simulink model "bpsk_receiver"  (R2020a)
settings: Solver=VariableStepAuto  StartTime=0.0  StopTime=10000/3.2e6  RelTol=1e-3
InitFcn:
  | setup_bpsk_receiver
undefined symbols (not defined in the file): AXI4, designMultirateFIR, fir_bbuf, Lite, tx_data, xlfda_numerator
libraries: xbsIndex_r4 x367, hdlsllib x15, dspmlti4 x8, xrbsSSR_Library x6, dspswit3 x4, dspsigops x2, commrandsrc3 x1, simulink x1
(part 3 of 4)

== system bpsk_receiver/Coarse Frequency Synchronisation/NCO ==
  Offset In : Inport
  AddSub : xbsIndex_r4/AddSub  mode=Addition  use_carryin=off  use_carryout=off  en=off  latency=0  precision=User Defined  arith_type=Unsigned  n_bits=41  bin_pt=41-10  quantization=Truncate  overflow=Wrap  use_behavioral_HDL=off  hw_selection=Fabric  pipelined=off  dbl_ovrd=off  block_type=addsub
  CMult : xbsIndex_r4/CMult  const=1024/(12.8e6)  gui_display_data_type=Fixed-point  const_n_bits=i+b  const_bin_pt=b  float_type=Single  exp_bits=8  fraction_bits=24  en=off  latency=1  precision=User Defined  arith_type="Signed  (2's comp)"  n_bits=n+b  bin_pt=b  quantization=Truncate  overflow=Saturate  use_behavioral_HDL=off  mem_type=Distributed RAM  pipeline=off  dbl_ovrd=off  block_type=cmult
  Convert4 : xbsIndex_r4/Convert  gui_display_data_type=Fixed-point  arith_type=Unsigned  n_bits=10  bin_pt=0  float_type=Single  exp_bits=8  fraction_bits=24  quantization=Truncate  overflow=Wrap  en=off  latency=0  pipeline=off  dbl_ovrd=off  block_type=convert
  Delay2 : xbsIndex_r4/Delay  rst=off  infoeditControl=Selection of Reset will increase slice count due to use of real FFs and instead of SRLs  en=off  latency=1  reg_retiming=off  dbl_ovrd=off  block_type=delay
  Sin_ROM : xbsIndex_r4/ROM  depth=1024  initVector=sin(pi*(0:1024-1)/(1024/2))  distributed_mem=Block RAM  rst=off  init_reg=0  en=off  latency=1  gui_display_data_type=Fixed-point  arith_type="Signed  (2's comp)"  n_bits=L  bin_pt=L-2  preci_type=Single  exp_width=8  frac_width=24  optimize=Area  use_rpm=on  dbl_ovrd=off  simulation_type=fast_sim  block_type=sprom
  cos_ROM : xbsIndex_r4/ROM  depth=1024  initVector=cos(pi*(0:1024-1)/(1024/2))  distributed_mem=Block RAM  rst=off  init_reg=0  en=off  latency=1  gui_display_data_type=Fixed-point  arith_type="Signed  (2's comp)"  n_bits=L  bin_pt=L-2  preci_type=Single  exp_width=8  frac_width=24  optimize=Area  use_rpm=on  dbl_ovrd=off  simulation_type=fast_sim  block_type=sprom
  cos : Outport  VectorParamsAs1DForOutWhenUnconnected=off
  sin : Outport  Port=2  VectorParamsAs1DForOutWhenUnconnected=off
  wires:
  cos_ROM/1 -> cos/1
  Sin_ROM/1 -> sin/1
  Convert4/1 -> cos_ROM/1, Sin_ROM/1
  CMult/1 -> AddSub/2
  Delay2/1 -> AddSub/1
  Offset In/1 -> CMult/1
  AddSub/1 -> Delay2/1, Convert4/1

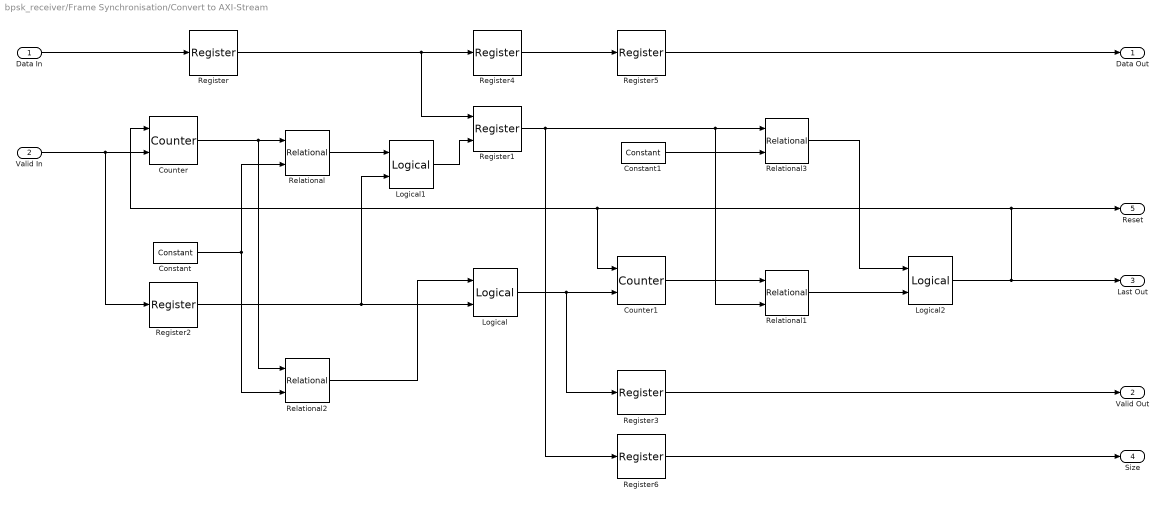
== system bpsk_receiver/Frame Synchronisation/Convert to AXI-Stream ==
  Data In : Inport
  Valid In : Inport  Port=2
  Constant : xbsIndex_r4/Constant  const=1.0  gui_display_data_type=Fixed-point  arith_type=Unsigned  n_bits=1  bin_pt=0  preci_type=Single  exp_width=8  frac_width=24  explicit_period=off  period=1  equ=P=C  opselect=C  inp2=PCIN>>17  opr=+  inp1=P  carry=CIN  dbl_ovrd=off  block_type=constant
  Constant1 : xbsIndex_r4/Constant  const=0  gui_display_data_type=Fixed-point  arith_type=Unsigned  n_bits=1  bin_pt=0  preci_type=Single  exp_width=8  frac_width=24  explicit_period=off  period=1  equ=P=C  opselect=C  inp2=PCIN>>17  opr=+  inp1=P  carry=CIN  dbl_ovrd=off  block_type=constant
  Counter : xbsIndex_r4/Counter  cnt_type=Free Running  cnt_to=Inf  operation=Up  start_count=0  cnt_by_val=1  arith_type=Unsigned  n_bits=32  bin_pt=0  load_pin=off  rst=on  en=on  explicit_period=off  period=1  use_behavioral_HDL=off  implementation=Fabric  dbl_ovrd=off  block_type=counter
  Counter1 : xbsIndex_r4/Counter  cnt_type=Free Running  cnt_to=Inf  operation=Up  start_count=0  cnt_by_val=1  arith_type=Unsigned  n_bits=32  bin_pt=0  load_pin=off  rst=on  en=on  explicit_period=off  period=1  use_behavioral_HDL=off  implementation=Fabric  dbl_ovrd=off  block_type=counter
  Logical : xbsIndex_r4/Logical  logical_function=AND  inputs=2  en=off  latency=1  precision=Full  arith_type=Unsigned  n_bits=16  bin_pt=0  align_bp=on  dbl_ovrd=off  block_type=logical
  Logical1 : xbsIndex_r4/Logical  logical_function=AND  inputs=2  en=off  latency=0  precision=Full  arith_type=Unsigned  n_bits=16  bin_pt=0  align_bp=on  dbl_ovrd=off  block_type=logical
  Logical2 : xbsIndex_r4/Logical  logical_function=AND  inputs=2  en=off  latency=0  precision=Full  arith_type=Unsigned  n_bits=16  bin_pt=0  align_bp=on  dbl_ovrd=off  block_type=logical
  Register{,2..6} (6 alike) : xbsIndex_r4/Register  init=0  rst=off  en=off  dbl_ovrd=off  block_type=register
  Register1 : xbsIndex_r4/Register  init=0  rst=off  en=on  dbl_ovrd=off  block_type=register
  Relational : xbsIndex_r4/Relational  mode=a=b  op_type=Bool  en=off  latency=0  dbl_ovrd=off  block_type=relational
  Relational1 : xbsIndex_r4/Relational  mode=a>=b  op_type=Bool  en=off  latency=0  dbl_ovrd=off  block_type=relational
  Relational2 : xbsIndex_r4/Relational  mode=a>b  op_type=Bool  en=off  latency=0  dbl_ovrd=off  block_type=relational
  Relational3 : xbsIndex_r4/Relational  mode=a!=b  op_type=Bool  en=off  latency=0  dbl_ovrd=off  block_type=relational
  Data Out : Outport  VectorParamsAs1DForOutWhenUnconnected=off
  Valid Out : Outport  Port=2  VectorParamsAs1DForOutWhenUnconnected=off
  Last Out : Outport  Port=3  VectorParamsAs1DForOutWhenUnconnected=off
  Size : Outport  Port=4  VectorParamsAs1DForOutWhenUnconnected=off
  Reset : Outport  Port=5  VectorParamsAs1DForOutWhenUnconnected=off
  wires:
  Register6/1 -> Size/1
  Logical2/1 -> Last Out/1, Reset/1, Counter1/1, Counter/1
  Relational1/1 -> Logical2/2
  Relational3/1 -> Logical2/1
  Constant1/1 -> Relational3/2
  Logical1/1 -> Register1/2
  Relational/1 -> Logical1/1
  Relational2/1 -> Logical/1
  Constant/1 -> Relational2/2, Relational/2
  Register5/1 -> Data Out/1
  Register4/1 -> Register5/1
  Register3/1 -> Valid Out/1
  Register2/1 -> Logical/2, Logical1/2
  Register1/1 -> Relational1/2, Relational3/1, Register6/1
  Counter1/1 -> Relational1/1
  Logical/1 -> Counter1/2, Register3/1
  Register/1 -> Register1/1, Register4/1
  Data In/1 -> Register/1
  Counter/1 -> Relational/1, Relational2/1
  Valid In/1 -> Counter/2, Register2/1

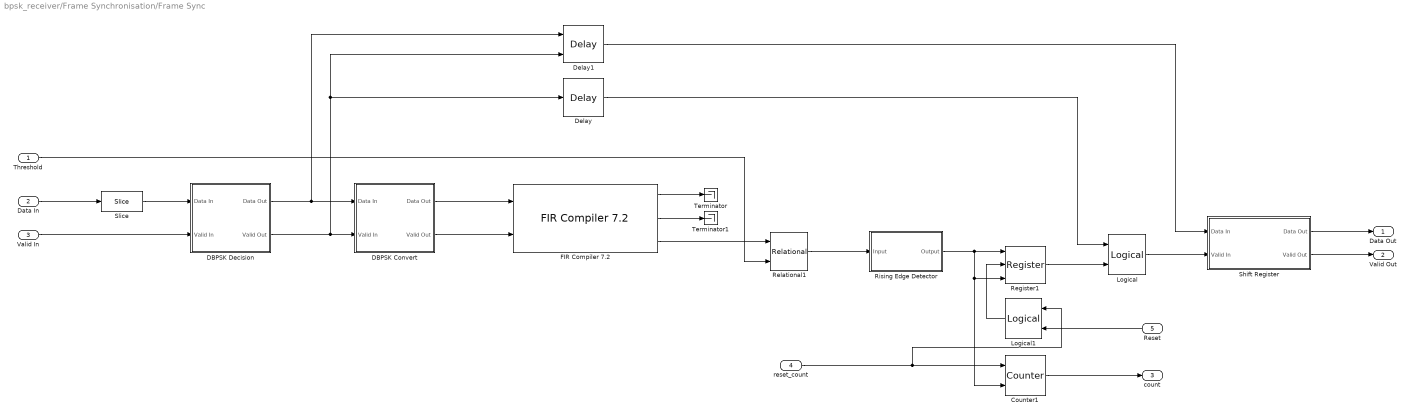
== system bpsk_receiver/Frame Synchronisation/Frame Sync ==
  Threshold : Inport
  Data In : Inport  Port=2
  Valid In : Inport  Port=3
  reset_count : Inport  Port=4
  Reset : Inport  Port=5
  Counter1 : xbsIndex_r4/Counter  cnt_type=Free Running  cnt_to=Inf  operation=Up  start_count=0  cnt_by_val=1  arith_type=Unsigned  n_bits=32  bin_pt=0  load_pin=off  rst=on  en=on  explicit_period=off  period=1  use_behavioral_HDL=off  implementation=Fabric  dbl_ovrd=off  block_type=counter
  DBPSK Convert : Subsystem
  DBPSK Decision : Subsystem
  Delay : xbsIndex_r4/Delay  rst=off  infoeditControl=Selection of Reset will increase slice count due to use of real FFs and instead of SRLs  en=off  latency=2  reg_retiming=off  dbl_ovrd=off  block_type=delay
  Delay1 : xbsIndex_r4/Delay  rst=off  infoeditControl=Selection of Reset will increase slice count due to use of real FFs and instead of SRLs  en=on  latency=2  reg_retiming=off  dbl_ovrd=off  block_type=delay
  "FIR Compiler 7.2 " : xbsIndex_r4/FIR Compiler 7.2   coefficientvector=fliplr(double(fir_bbuf))  coefficient_sets=1  coefficient_reload=off  filter_type=Single_Rate  rate_change_type=Integer  interpolation_rate=1  decimation_rate=1  zero_pack_factor=1  channel_sequence=Basic  number_channels=1  pattern_list='P4-0,P4-1,P4-2,P4-3,P4-4'  number_paths=1  ratespecification=Maximum_Possible  sampleperiod=40  hardwareoversamplingrate=1  coefficient_sign=Signed  quantization=Integer_Coefficients  coefficient_width=2  bestprecision=off  coefficient_fractional_bits=0  coefficient_structure=Inferred  output_rounding_mode=Full_Precision  output_width=22  filter_architecture=Systolic_Multiply_Accumulate  optimization_goal=Area  optimization_list='None'  data_buffer_type=Automatic  coefficient_buffer_type=Automatic  input_buffer_type=Automatic  output_buffer_type=Automatic  preference_for_other_storage=Automatic  multi_column_support=Automatic  columnconfig='39'  inter_column_pipe_length=4  data_has_tlast=Not_Required  m_data_has_tready=off  s_data_has_fifo=off  s_data_has_tuser=Not_Required  m_data_has_tuser=Not_Required  s_config_sync_mode=On_Vector  s_config_method=Single  num_reload_slots=1  has_aclken=on  has_aresetn=off  infoeditControl=ARESETn must be asserted for a minimum of 2 cycles  reset_data_vector=on  trim_axipin_name=on  simulation_type=hybrid_sim  simulation_model=sysgen:xfirv7_2_cmodel  data_path_portlist={ 's_axis_data_tdata', 'm_axis_data_tdata' }  passband_min=0.0  passband_max=0.5  stopband_min=0.5  stopband_max=1.0  filter_selection=1  gui_behaviour='Sysgen_GUI'  data_sign=Signed  data_width=16  data_fractional_bits=0  data_tuser_width=1  wrapper_available=true  ip_wrap_arbitrary_binary_point=true  ip_name=FIR Compiler  ip_version=7.2  dsptool_ready=true  ipcore_usecache=true  ipcore_useipmodelcache=true  port_translation_map={ 'aclken' => 'en', 'aresetn' => 'rst' }  run_core_at_system_period=true  ipcore_xco_need_fpga_part=true  block_type=fir_compiler_v7_2
      settings: infoedit=Maximum Possible : Maximizes oversampling rate. Abstracted input handshake (no s_data_tvalid) and automatic rate propagation.<br>Hardware Oversampling Rate : Specifies oversampling rate relative to the input sample period. Abstracted input handshake (no s_data_tvalid) and automatic rate propagation.<br>Input/Output Sample Period : Specifies absolute oversampling rate. No input handshake abstraction (exposes s_data_tvalid) and no rate propagation.
  Logical : xbsIndex_r4/Logical  logical_function=AND  inputs=2  en=off  latency=0  precision=Full  arith_type=Unsigned  n_bits=16  bin_pt=0  align_bp=on  dbl_ovrd=off  block_type=logical
  Logical1 : xbsIndex_r4/Logical  logical_function=OR  inputs=2  en=off  latency=0  precision=Full  arith_type=Unsigned  n_bits=16  bin_pt=0  align_bp=on  dbl_ovrd=off  block_type=logical
  Register1 : xbsIndex_r4/Register  init=0  rst=on  en=on  dbl_ovrd=off  block_type=register
  Relational1 : xbsIndex_r4/Relational  mode=a>=b  op_type=Bool  en=off  latency=0  dbl_ovrd=off  block_type=relational
  Rising Edge Detector : Subsystem
  Shift Register : Subsystem
  Slice : xbsIndex_r4/Slice  nbits=1  boolean_output=off  mode=Upper Bit Location + Width  bit1=0  base1=MSB of Input  bit0=0  base0=LSB of Input  dbl_ovrd=off  block_type=slice
  Terminator : Terminator
  Terminator1 : Terminator
  Data Out : Outport  VectorParamsAs1DForOutWhenUnconnected=off
  Valid Out : Outport  Port=2  VectorParamsAs1DForOutWhenUnconnected=off
  count : Outport  Port=3  VectorParamsAs1DForOutWhenUnconnected=off
  wires:
  Shift Register/2(Valid Out) -> Valid Out/1
  Data In/1 -> Slice/1
  Delay/1 -> Logical/1
  "FIR Compiler 7.2 "/3 -> Relational1/1
  reset_count/1 -> Counter1/1, Logical1/1
  "FIR Compiler 7.2 "/1 -> Terminator/1
  DBPSK Convert/2(Valid Out) -> "FIR Compiler 7.2 "/2
  Shift Register/1(Data Out) -> Data Out/1
  Register1/1 -> Logical/2
  Rising Edge Detector/1(Output) -> Register1/1, Register1/3, Counter1/2
  "FIR Compiler 7.2 "/2 -> Terminator1/1
  Slice/1 -> DBPSK Decision/1(Data In)
  Valid In/1 -> DBPSK Decision/2(Valid In)
  Counter1/1 -> count/1
  Logical1/1 -> Register1/2
  Threshold/1 -> Relational1/2
  Logical/1 -> Shift Register/2(Valid In)
  Delay1/1 -> Shift Register/1(Data In)
  DBPSK Decision/1(Data Out) -> DBPSK Convert/1(Data In), Delay1/1
  Relational1/1 -> Rising Edge Detector/1(Input)
  Reset/1 -> Logical1/2
  DBPSK Decision/2(Valid Out) -> DBPSK Convert/2(Valid In), Delay/1, Delay1/2
  DBPSK Convert/1(Data Out) -> "FIR Compiler 7.2 "/1

== system bpsk_receiver/Observation Point/op ==
  Data In : Inport
  Valid In : Inport  Port=2
  Cast To Boolean : DataTypeConversion  OutDataTypeStr=boolean
  Constellation Diagram : ConstellationDiagram
  Convert Protect : DataTypeConversion  OutDataTypeStr=fixdt(0,32,0)  ConvertRealWorld=Stored Integer (SI)
  Delay : Delay  DelayLength=1  ShowEnablePort=on
      settings: InputPortMap=u0,e6
  Imag Conversion : DataTypeConversion  OutDataTypeStr=fixdt(1,16,15)  ConvertRealWorld=Stored Integer (SI)
  Imag Slice : hdlsllib/Logic and Bit Operations/Bit Slice  lidx=31  ridx=16
      settings: SourceProductBaseCode=SL
  Real Conversion : DataTypeConversion  OutDataTypeStr=fixdt(1,16,15)  ConvertRealWorld=Stored Integer (SI)
  Real Slice : hdlsllib/Logic and Bit Operations/Bit Slice  lidx=15  ridx=0
      settings: SourceProductBaseCode=SL
  Real-Imag to Complex : RealImagToComplex
  Time Scope : Scope
  m_axis_op_tdata : xbsIndex_r4/Gateway Out  inherit_from_input=on  hdl_port=on  rows=1  columns=1  UseAsDAC=off  DACChannel='1'  interface=None  automatic_assignment=on  address_offset=hex2dec('00')  intf_name=''  intf_description=''  timing_constraint=None  locs_specified=off  LOCs={}  io_standard={}  block_type=gatewayout
  m_axis_op_tvalid : xbsIndex_r4/Gateway Out  inherit_from_input=on  hdl_port=on  rows=1  columns=1  UseAsDAC=off  DACChannel='1'  interface=None  automatic_assignment=on  address_offset=hex2dec('00')  intf_name=''  intf_description=''  timing_constraint=None  locs_specified=off  LOCs={}  io_standard={}  block_type=gatewayout
  wires:
  Cast To Boolean/1 -> Delay/2
  Convert Protect/1 -> Imag Slice/1, Real Slice/1
  Real-Imag to Complex/1 -> Delay/1
  m_axis_op_tdata/1 -> Convert Protect/1
  Imag Conversion/1 -> Real-Imag to Complex/2
  Imag Slice/1 -> Imag Conversion/1
  Real Slice/1 -> Real Conversion/1
  Real Conversion/1 -> Real-Imag to Complex/1
  m_axis_op_tvalid/1 -> Cast To Boolean/1
  Delay/1 -> Constellation Diagram/1, Time Scope/1
  Data In/1 -> m_axis_op_tdata/1
  Valid In/1 -> m_axis_op_tvalid/1

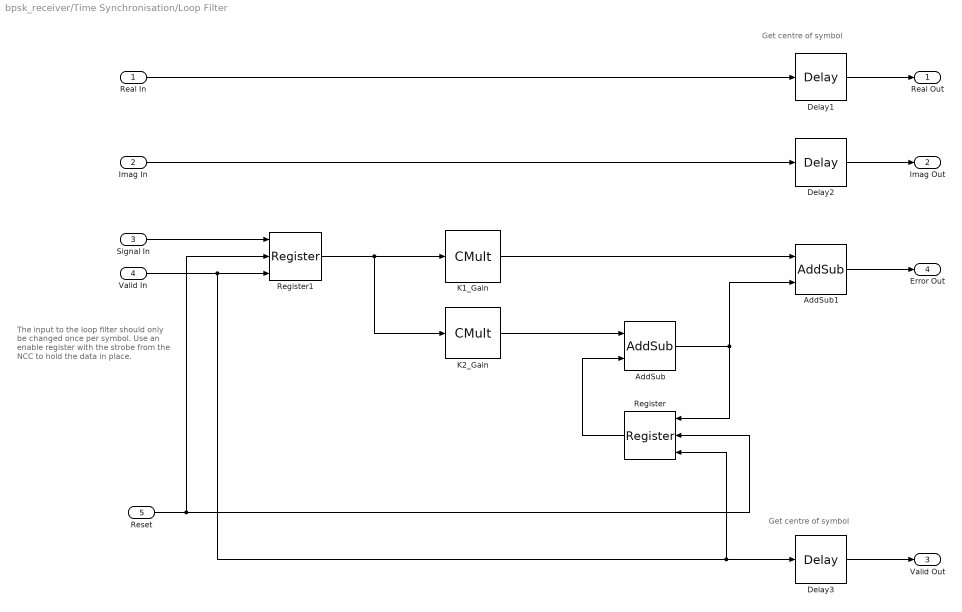
== system bpsk_receiver/Time Synchronisation/Loop Filter ==
  note: Get centre of symbol
  note: The input to the loop filter should only be changed once per symbol.
      |
      | Use an enable register with the strobe from the NCC to hold the data in place.
  note: Get centre of symbol
  Real In : Inport
  Imag In : Inport  Port=2
  Signal In : Inport  Port=3
  Valid In : Inport  Port=4
  Reset : Inport  Port=5
  AddSub : xbsIndex_r4/AddSub  mode=Addition  use_carryin=off  use_carryout=off  en=off  latency=0  precision=User Defined  arith_type="Signed  (2's comp)"  n_bits=64  bin_pt=60  quantization=Truncate  overflow=Saturate  use_behavioral_HDL=off  hw_selection=Fabric  pipelined=off  dbl_ovrd=off  block_type=addsub
  AddSub1 : xbsIndex_r4/AddSub  mode=Addition  use_carryin=off  use_carryout=off  en=off  latency=0  precision=User Defined  arith_type="Signed  (2's comp)"  n_bits=64  bin_pt=60  quantization=Truncate  overflow=Saturate  use_behavioral_HDL=off  hw_selection=Fabric  pipelined=off  dbl_ovrd=off  block_type=addsub
  Delay1 : xbsIndex_r4/Delay  rst=off  infoeditControl=Selection of Reset will increase slice count due to use of real FFs and instead of SRLs  en=off  latency=32/2  reg_retiming=off  dbl_ovrd=off  block_type=delay
  Delay2 : xbsIndex_r4/Delay  rst=off  infoeditControl=Selection of Reset will increase slice count due to use of real FFs and instead of SRLs  en=off  latency=32/2  reg_retiming=off  dbl_ovrd=off  block_type=delay
  Delay3 : xbsIndex_r4/Delay  rst=off  infoeditControl=Selection of Reset will increase slice count due to use of real FFs and instead of SRLs  en=off  latency=32/2  reg_retiming=off  dbl_ovrd=off  block_type=delay
  K1_Gain : xbsIndex_r4/CMult  const=K1  gui_display_data_type=Fixed-point  const_n_bits=32  const_bin_pt=30  float_type=Single  exp_bits=8  fraction_bits=24  en=off  latency=0  precision=Full  arith_type="Signed  (2's comp)"  n_bits=3+28+16  bin_pt=28+16  quantization=Truncate  overflow=Wrap  use_behavioral_HDL=off  mem_type=Distributed RAM  pipeline=off  dbl_ovrd=off  block_type=cmult
  K2_Gain : xbsIndex_r4/CMult  const=K2  gui_display_data_type=Fixed-point  const_n_bits=32  const_bin_pt=30  float_type=Single  exp_bits=8  fraction_bits=24  en=off  latency=0  precision=Full  arith_type="Signed  (2's comp)"  n_bits=3+28+16  bin_pt=28+16  quantization=Truncate  overflow=Wrap  use_behavioral_HDL=off  mem_type=Distributed RAM  pipeline=off  dbl_ovrd=off  block_type=cmult
  Register : xbsIndex_r4/Register  init=0  rst=on  en=on  dbl_ovrd=off  block_type=register
  Register1 : xbsIndex_r4/Register  init=0  rst=on  en=on  dbl_ovrd=off  block_type=register
  Real Out : Outport  VectorParamsAs1DForOutWhenUnconnected=off
  Imag Out : Outport  Port=2  VectorParamsAs1DForOutWhenUnconnected=off
  Valid Out : Outport  Port=3  VectorParamsAs1DForOutWhenUnconnected=off
  Error Out : Outport  Port=4  VectorParamsAs1DForOutWhenUnconnected=off
  wires:
  AddSub1/1 -> Error Out/1
  Valid In/1 -> Register1/3, Delay3/1, Register/3
  Delay1/1 -> Real Out/1
  Delay2/1 -> Imag Out/1
  Register1/1 -> K2_Gain/1, K1_Gain/1
  Signal In/1 -> Register1/1
  Register/1 -> AddSub/2
  K1_Gain/1 -> AddSub1/1
  AddSub/1 -> AddSub1/2, Register/1
  Imag In/1 -> Delay2/1
  Real In/1 -> Delay1/1
  K2_Gain/1 -> AddSub/1
  Reset/1 -> Register1/2, Register/2
  Delay3/1 -> Valid Out/1

== system bpsk_receiver/Time Synchronisation/NCC ==
  Error : Inport
  AddSub : xbsIndex_r4/AddSub  mode=Addition  use_carryin=off  use_carryout=off  en=off  latency=0  precision=User Defined  arith_type=Unsigned  n_bits=n+f  bin_pt=f  quantization=Truncate  overflow=Wrap  use_behavioral_HDL=off  hw_selection=Fabric  pipelined=off  dbl_ovrd=off  block_type=addsub
  AddSub1 : xbsIndex_r4/AddSub  mode=Addition  use_carryin=off  use_carryout=off  en=off  latency=0  precision=User Defined  arith_type="Signed  (2's comp)"  n_bits=n+f  bin_pt=f  quantization=Truncate  overflow=Saturate  use_behavioral_HDL=off  hw_selection=Fabric  pipelined=off  dbl_ovrd=off  block_type=addsub
  AddSub2 : xbsIndex_r4/AddSub  mode=Subtraction  use_carryin=off  use_carryout=off  en=off  latency=0  precision=User Defined  arith_type="Signed  (2's comp)"  n_bits=n+f  bin_pt=f  quantization=Truncate  overflow=Flag as error  use_behavioral_HDL=off  hw_selection=Fabric  pipelined=off  dbl_ovrd=off  block_type=addsub
  Constant : xbsIndex_r4/Constant  const=1  gui_display_data_type=Fixed-point  arith_type=Unsigned  n_bits=1  bin_pt=0  preci_type=Single  exp_width=8  frac_width=24  explicit_period=off  period=1  equ=P=C  opselect=C  inp2=PCIN>>17  opr=+  inp1=P  carry=CIN  dbl_ovrd=off  block_type=constant
  Constant1 : xbsIndex_r4/Constant  const=r  gui_display_data_type=Fixed-point  arith_type=Unsigned  n_bits=n  bin_pt=0  preci_type=Single  exp_width=8  frac_width=24  explicit_period=off  period=1  equ=P=C  opselect=C  inp2=PCIN>>17  opr=+  inp1=P  carry=CIN  dbl_ovrd=off  block_type=constant
  Mux : xbsIndex_r4/Mux  inputs=2  en=off  latency=0  precision=Full  arith_type=Unsigned  n_bits=16  bin_pt=14  quantization=Truncate  overflow=Wrap  dbl_ovrd=off  block_type=mux
  Register : xbsIndex_r4/Register  init=0  rst=off  en=off  dbl_ovrd=off  block_type=register
  Relational : xbsIndex_r4/Relational  mode=a>b  op_type=Bool  en=off  latency=0  dbl_ovrd=off  block_type=relational
  Relational1 : xbsIndex_r4/Relational  mode=a>b  op_type=Bool  en=off  latency=0  dbl_ovrd=off  block_type=relational
  Strobe : Outport  VectorParamsAs1DForOutWhenUnconnected=off
  wires:
  Mux/1 -> AddSub/1
  Relational1/1 -> Mux/1
  AddSub2/1 -> Mux/3
  Constant1/1 -> Relational1/2, AddSub2/2
  Register/1 -> Relational/1, Relational1/1, Mux/2, AddSub2/1
  AddSub/1 -> Register/1, Relational/2
  Relational/1 -> Strobe/1
  Error/1 -> AddSub1/2
  Constant/1 -> AddSub1/1
  AddSub1/1 -> AddSub/2

== system bpsk_receiver/Time Synchronisation/Timing Error Detector ==
  Real In : Inport
  Imag In : Inport  Port=2
  AddSub : xbsIndex_r4/AddSub  mode=Subtraction  use_carryin=off  use_carryout=off  en=off  latency=0  precision=User Defined  arith_type="Signed  (2's comp)"  n_bits=31  bin_pt=30  quantization=Truncate  overflow=Saturate  use_behavioral_HDL=off  hw_selection=Fabric  pipelined=off  dbl_ovrd=off  block_type=addsub
  AddSub1 : xbsIndex_r4/AddSub  mode=Subtraction  use_carryin=off  use_carryout=off  en=off  latency=0  precision=User Defined  arith_type="Signed  (2's comp)"  n_bits=31  bin_pt=30  quantization=Truncate  overflow=Saturate  use_behavioral_HDL=off  hw_selection=Fabric  pipelined=off  dbl_ovrd=off  block_type=addsub
  AddSub2 : xbsIndex_r4/AddSub  mode=Addition  use_carryin=off  use_carryout=off  en=off  latency=0  precision=Full  arith_type="Signed  (2's comp)"  n_bits=16  bin_pt=13  quantization="Round  (unbiased: +/- Inf)"  overflow=Saturate  use_behavioral_HDL=off  hw_selection=Fabric  pipelined=off  dbl_ovrd=off  block_type=addsub
  CMult : xbsIndex_r4/CMult  const=10  gui_display_data_type=Fixed-point  const_n_bits=4  const_bin_pt=0  float_type=Single  exp_bits=8  fraction_bits=24  en=off  latency=0  precision=User Defined  arith_type="Signed  (2's comp)"  n_bits=32  bin_pt=30  quantization=Truncate  overflow=Saturate  use_behavioral_HDL=off  mem_type=Distributed RAM  pipeline=off  dbl_ovrd=off  block_type=cmult
  Delay : xbsIndex_r4/Delay  rst=off  infoeditControl=Selection of Reset will increase slice count due to use of real FFs and instead of SRLs  en=off  latency=32  reg_retiming=off  dbl_ovrd=off  block_type=delay
  Delay1 : xbsIndex_r4/Delay  rst=off  infoeditControl=Selection of Reset will increase slice count due to use of real FFs and instead of SRLs  en=off  latency=32  reg_retiming=off  dbl_ovrd=off  block_type=delay
  Mult1 : xbsIndex_r4/Mult  precision=User Defined  arith_type=Unsigned  n_bits=31  bin_pt=30  quantization=Truncate  overflow=Saturate  en=off  latency=0  use_behavioral_HDL=off  opt=Speed  use_embedded=on  optimum_pipeline=off  pipeline=on  dbl_ovrd=off  use_rpm=on  placement_style=Triangular  block_type=mult
  Mult2 : xbsIndex_r4/Mult  precision=User Defined  arith_type=Unsigned  n_bits=31  bin_pt=30  quantization=Truncate  overflow=Saturate  en=off  latency=0  use_behavioral_HDL=off  opt=Speed  use_embedded=on  optimum_pipeline=off  pipeline=on  dbl_ovrd=off  use_rpm=on  placement_style=Triangular  block_type=mult
  Reinterpret : xbsIndex_r4/Reinterpret  force_arith_type=on  arith_type="Signed  (2's comp)"  force_bin_pt=on  bin_pt=15  block_type=reinterpret
  Reinterpret1 : xbsIndex_r4/Reinterpret  force_arith_type=on  arith_type="Signed  (2's comp)"  force_bin_pt=on  bin_pt=15  block_type=reinterpret
  Error : Outport  VectorParamsAs1DForOutWhenUnconnected=off
  wires:
  Reinterpret1/1 -> Mult1/2, Mult1/1
  Reinterpret/1 -> Mult2/1, Mult2/2
  Delay/1 -> AddSub/2
  Mult1/1 -> Delay/1, AddSub/1
  AddSub1/1 -> AddSub2/2
  Mult2/1 -> AddSub1/1, Delay1/1
  Delay1/1 -> AddSub1/2
  AddSub2/1 -> CMult/1
  AddSub/1 -> AddSub2/1
  Imag In/1 -> Reinterpret/1
  Real In/1 -> Reinterpret1/1
  CMult/1 -> Error/1

== system bpsk_receiver/BPSK System/BPSK TX Generation/DBPSK Modulator ==
  Input : Inport
  Cast To Boolean : DataTypeConversion  OutDataTypeStr=boolean
  Constant : Constant  Value=fi(1, 1, 16, 14)  OutDataTypeStr=fixdt(1,16,14)  SampleTime=-1
  Constant1 : Constant  Value=fi(-1, 1, 16, 14)  OutDataTypeStr=fixdt(1,16,14)  SampleTime=-1
  Constant2 : Constant  Value=0  OutDataTypeStr=Inherit: Inherit via back propagation  SampleTime=-1
  Delay : Delay  DelayLength=1
  Multiport Switch : MultiPortSwitch  DataPortOrder=Zero-based contiguous  Inputs=2  zeroidx=on
  Real-Imag to Complex : RealImagToComplex
  XOR : Logic  Operator=XOR  IconShape=distinctive  AllPortsSameDT=off  OutDataTypeStr=boolean
  Output : Outport  VectorParamsAs1DForOutWhenUnconnected=off
  wires:
  Cast To Boolean/1 -> XOR/2
  XOR/1 -> Delay/1, Multiport Switch/1
  Delay/1 -> XOR/1
  Input/1 -> Cast To Boolean/1
  Constant/1 -> Multiport Switch/2
  Constant1/1 -> Multiport Switch/3
  Multiport Switch/1 -> Real-Imag to Complex/1
  Real-Imag to Complex/1 -> Output/1
  Constant2/1 -> Real-Imag to Complex/2

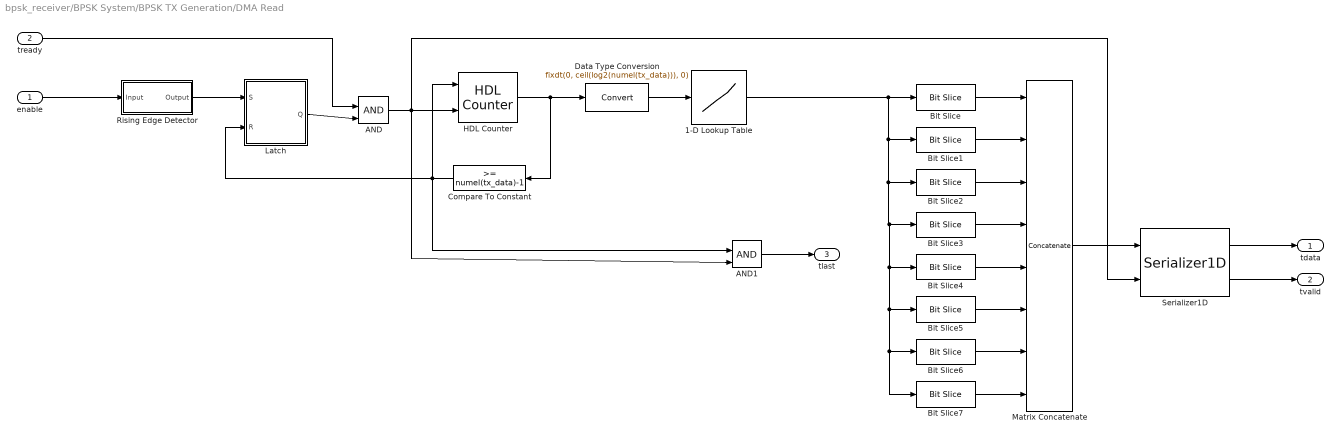
== system bpsk_receiver/BPSK System/BPSK TX Generation/DMA Read ==
  enable : Inport
  tready : Inport  Port=2
  1-D Lookup Table : Lookup_n-D  NumberOfTableDimensions=1  BreakpointsForDimension1=[0:1:numel(tx_data)-1]  Table=tx_data  TableDataTypeStr=Inherit: Inherit from 'Table data'  ExtrapMethod=Clip  InternalRulePriority=Speed  OutDataTypeStr=Inherit: Inherit from 'Table data'  RndMeth=Simplest  InputSameDT=on
  AND : Logic  IconShape=distinctive  AllPortsSameDT=off  OutDataTypeStr=boolean
  AND1 : Logic  IconShape=distinctive  AllPortsSameDT=off  OutDataTypeStr=boolean
  Bit Slice : hdlsllib/Logic and Bit Operations/Bit Slice  lidx=0  ridx=0
      settings: SourceProductBaseCode=SL
  Bit Slice1 : hdlsllib/Logic and Bit Operations/Bit Slice  lidx=1  ridx=1
      settings: SourceProductBaseCode=SL
  Bit Slice2 : hdlsllib/Logic and Bit Operations/Bit Slice  lidx=2  ridx=2
      settings: SourceProductBaseCode=SL
  Bit Slice3 : hdlsllib/Logic and Bit Operations/Bit Slice  lidx=3  ridx=3
      settings: SourceProductBaseCode=SL
  Bit Slice4 : hdlsllib/Logic and Bit Operations/Bit Slice  lidx=4  ridx=4
      settings: SourceProductBaseCode=SL
  Bit Slice5 : hdlsllib/Logic and Bit Operations/Bit Slice  lidx=5  ridx=5
      settings: SourceProductBaseCode=SL
  Bit Slice6 : hdlsllib/Logic and Bit Operations/Bit Slice  lidx=6  ridx=6
      settings: SourceProductBaseCode=SL
  Bit Slice7 : hdlsllib/Logic and Bit Operations/Bit Slice  lidx=7  ridx=7
      settings: SourceProductBaseCode=SL
  Compare To Constant : simulink/Logic and Bit Operations/Compare To Constant  relop=>=  const=numel(tx_data)-1  OutDataTypeStr=boolean
  Data Type Conversion : DataTypeConversion  OutDataTypeStr=fixdt(0, ceil(log2(numel(tx_data))), 0)
  HDL Counter : hdlsllib/Sources/HDL Counter  CountType=Free running  CountInit=0  CountStep=1  CountMax=25  CountFromType=Initial value  CountFrom=0  CountResetPort=on  CountLoadPort=off  CountEnbPort=on  CountDirPort=off  CountDataType=Unsigned  CountWordLen=32  CountFracLen=0  CountSampTime=1
  Latch : Subsystem
  Matrix Concatenate : Concatenate  NumInputs=8  Mode=Multidimensional array  ConcatenateDimension=2
  Rising Edge Detector : Subsystem
  Serializer1D : hdlsllib/HDL Operations/Serializer1D  Ratio=8  IdleCycles=0  validIn=on  startOut=off  validOut=on  inputDataDimensions=-1  inputSampleTime=-1  inputSignalType=auto
      settings: SourceProductBaseCode=SL
  tdata : Outport  VectorParamsAs1DForOutWhenUnconnected=off
  tvalid : Outport  Port=2  VectorParamsAs1DForOutWhenUnconnected=off
  tlast : Outport  Port=3  VectorParamsAs1DForOutWhenUnconnected=off
  wires:
  AND1/1 -> tlast/1
  tready/1 -> AND/1
  Latch/1(Q) -> AND/2
  AND/1 -> HDL Counter/2, Serializer1D/2, AND1/2
  Rising Edge Detector/1(Output) -> Latch/1(S)
  Data Type Conversion/1 -> 1-D Lookup Table/1
  HDL Counter/1 -> Data Type Conversion/1, Compare To Constant/1
  enable/1 -> Rising Edge Detector/1(Input)
  Compare To Constant/1 -> Latch/2(R), HDL Counter/1, AND1/1
  Matrix Concatenate/1 -> Serializer1D/1
  Bit Slice/1 -> Matrix Concatenate/1
  Bit Slice3/1 -> Matrix Concatenate/4
  Bit Slice1/1 -> Matrix Concatenate/2
  Bit Slice2/1 -> Matrix Concatenate/3
  1-D Lookup Table/1 -> Bit Slice7/1, Bit Slice6/1, Bit Slice5/1, Bit Slice4/1, Bit Slice3/1, Bit Slice2/1, Bit Slice1/1, Bit Slice/1
  Serializer1D/1 -> tdata/1
  Bit Slice4/1 -> Matrix Concatenate/5
  Bit Slice7/1 -> Matrix Concatenate/8
  Bit Slice6/1 -> Matrix Concatenate/7
  Bit Slice5/1 -> Matrix Concatenate/6
  Serializer1D/2 -> tvalid/1

== system bpsk_receiver/BPSK System/RF-ADC/Decimation Filter ==
  Data In : Inport
  FIR 0 : dspmlti4/FIR Decimation  FilterSource=Filter object  h=designMultirateFIR(1,2)  D=2  filtStruct=Direct form  FilterObject=fir0  InputProcessing=Columns as channels (frame based)  framing=Allow multirate processing  inputOffset=0  outputBufInitCond=0  roundingMode=Floor  overflowMode=off  firstCoeffDataTypeStr=Inherit: Same word length as input  firstCoeffMin=[]  firstCoeffMax=[]  firstCoeffLastDataTypeStr=Inherit: Same word length as input  outputDataTypeStr=Inherit: Same as accumulator  outputMin=[]  outputMax=[]  outputLastDataTypeStr=Inherit: Same as accumulator
  FIR 1 : dspmlti4/FIR Decimation  FilterSource=Filter object  h=designMultirateFIR(1,2)  D=2  filtStruct=Direct form  FilterObject=fir1  InputProcessing=Columns as channels (frame based)  framing=Allow multirate processing  inputOffset=0  outputBufInitCond=0  roundingMode=Floor  overflowMode=off  firstCoeffDataTypeStr=Inherit: Same word length as input  firstCoeffMin=[]  firstCoeffMax=[]  firstCoeffLastDataTypeStr=Inherit: Same word length as input  outputDataTypeStr=Inherit: Same as accumulator  outputMin=[]  outputMax=[]  outputLastDataTypeStr=Inherit: Same as accumulator
  FIR 2 : dspmlti4/FIR Decimation  FilterSource=Filter object  h=designMultirateFIR(1,2)  D=2  filtStruct=Direct form  FilterObject=fir2  InputProcessing=Columns as channels (frame based)  framing=Allow multirate processing  inputOffset=0  outputBufInitCond=0  roundingMode=Floor  overflowMode=off  firstCoeffDataTypeStr=Inherit: Same word length as input  firstCoeffMin=[]  firstCoeffMax=[]  firstCoeffLastDataTypeStr=Inherit: Same word length as input  outputDataTypeStr=Inherit: Same as accumulator  outputMin=[]  outputMax=[]  outputLastDataTypeStr=Inherit: Same as accumulator
  Data Out : Outport  VectorParamsAs1DForOutWhenUnconnected=off
  wires:
  FIR 1/1 -> FIR 0/1
  FIR 0/1 -> Data Out/1
  Data In/1 -> FIR 2/1
  FIR 2/1 -> FIR 1/1

== system bpsk_receiver/BPSK System/RF-ADC/NCO and Mixer ==
  Data In : Inport
  Constant1 : Constant  Value=m  OutDataTypeStr=fixdt(0,2,0)  SampleTime=-1
  Data Type Conversion : DataTypeConversion  OutDataTypeStr=fixdt(1,16,14)
  Multiport Switch1 : MultiPortSwitch  DataPortOrder=Zero-based contiguous  zeroidx=on
  RF-ADC Coarse Mixer : Subsystem
  RF-ADC Fine Mixer : Subsystem
  Real-Imag to Complex : RealImagToComplex
  Data Out : Outport  VectorParamsAs1DForOutWhenUnconnected=off
  wires:
  Multiport Switch1/1 -> Data Out/1
  RF-ADC Fine Mixer/1(Data Out) -> Multiport Switch1/4
  Real-Imag to Complex/1 -> Data Type Conversion/1
  RF-ADC Coarse Mixer/1(Data Out) -> Multiport Switch1/3
  Data In/1 -> Real-Imag to Complex/1, RF-ADC Coarse Mixer/1(Data In), RF-ADC Fine Mixer/1(Data In), Real-Imag to Complex/2
  Constant1/1 -> Multiport Switch1/1
  Data Type Conversion/1 -> Multiport Switch1/2

== system bpsk_receiver/BPSK System/RF-ADC/RF-ADC ==
  Data In : Inport
  Buffer : Buffer  N=ssr  OutputFrames=off
  Data Type Conversion : DataTypeConversion  OutDataTypeStr=fixdt(1,12,10)
  Rate Transition : RateTransition  OutPortSampleTime=1/fs
  Data Out : Outport  VectorParamsAs1DForOutWhenUnconnected=off
  wires:
  Rate Transition/1 -> Data Type Conversion/1
  Data In/1 -> Rate Transition/1
  Data Type Conversion/1 -> Buffer/1
  Buffer/1 -> Data Out/1

== system bpsk_receiver/BPSK System/RF-DAC/Coarse Delay ==
  Data In : Inport
  Data Out : Outport  VectorParamsAs1DForOutWhenUnconnected=off
  wires:
  Data In/1 -> Data Out/1

== system bpsk_receiver/BPSK System/RF-DAC/Interpolation Filter ==
  Data In : Inport
  FIR 0 : dspmlti4/FIR Interpolation  FilterSource=Filter object  PrivateCoeffs=0  h=designMultirateFIR(3,1)  L=2  FilterObject=fir0  InputProcessing=Columns as channels (frame based)  framing=Allow multirate processing  outputBufInitCond=0  roundingMode=Floor  overflowMode=off  firstCoeffDataTypeStr=Inherit: Same word length as input  firstCoeffMin=[]  firstCoeffMax=[]  firstCoeffLastDataTypeStr=Inherit: Same word length as input  outputDataTypeStr=Inherit: Same as accumulator  outputMin=[]  outputMax=[]  outputLastDataTypeStr=Inherit: Same as accumulator
  FIR 1 : dspmlti4/FIR Interpolation  FilterSource=Filter object  PrivateCoeffs=0  h=designMultirateFIR(3,1)  L=2  FilterObject=fir1  InputProcessing=Columns as channels (frame based)  framing=Allow multirate processing  outputBufInitCond=0  roundingMode=Floor  overflowMode=off  firstCoeffDataTypeStr=Inherit: Same word length as input  firstCoeffMin=[]  firstCoeffMax=[]  firstCoeffLastDataTypeStr=Inherit: Same word length as input  outputDataTypeStr=Inherit: Same as accumulator  outputMin=[]  outputMax=[]  outputLastDataTypeStr=Inherit: Same as accumulator
  FIR 2 : dspmlti4/FIR Interpolation  FilterSource=Filter object  PrivateCoeffs=0  h=designMultirateFIR(3,1)  L=2  FilterObject=fir2  InputProcessing=Columns as channels (frame based)  framing=Allow multirate processing  outputBufInitCond=0  roundingMode=Floor  overflowMode=off  firstCoeffDataTypeStr=Inherit: Same word length as input  firstCoeffMin=[]  firstCoeffMax=[]  firstCoeffLastDataTypeStr=Inherit: Same word length as input  outputDataTypeStr=Inherit: Same as accumulator  outputMin=[]  outputMax=[]  outputLastDataTypeStr=Inherit: Same as accumulator
  Data Out : Outport  VectorParamsAs1DForOutWhenUnconnected=off
  wires:
  FIR 2/1 -> FIR 1/1
  Data In/1 -> FIR 2/1
  FIR 0/1 -> Data Out/1
  FIR 1/1 -> FIR 0/1

== system bpsk_receiver/BPSK System/RF-DAC/NCO and Mixer ==
  Data In : Inport
  Complex to Real-Imag : ComplexToRealImag
  Constant1 : Constant  Value=m  OutDataTypeStr=fixdt(0,2,0)  SampleTime=-1
  Multiport Switch1 : MultiPortSwitch  DataPortOrder=Zero-based contiguous  zeroidx=on
  RF-DAC Coarse Mixer : Subsystem
  RF-DAC Fine Mixer : Subsystem
  Terminator : Terminator
  Data Out : Outport  VectorParamsAs1DForOutWhenUnconnected=off
  wires:
  RF-DAC Coarse Mixer/1(Data Out) -> Multiport Switch1/3
  Constant1/1 -> Multiport Switch1/1
  Data In/1 -> Complex to Real-Imag/1, RF-DAC Coarse Mixer/1(Data In), RF-DAC Fine Mixer/1(Data In)
  Multiport Switch1/1 -> Data Out/1
  RF-DAC Fine Mixer/1(Data Out) -> Multiport Switch1/4
  Complex to Real-Imag/1 -> Multiport Switch1/2
  Complex to Real-Imag/2 -> Terminator/1

== system bpsk_receiver/BPSK System/RF-DAC/Output Filter ==
  Data In : Inport
  Data Out : Outport  VectorParamsAs1DForOutWhenUnconnected=off
  wires:
  Data In/1 -> Data Out/1

== system bpsk_receiver/BPSK System/RF-DAC/QMC Gain & Phase ==
  Data In : Inport
  Data Out : Outport  VectorParamsAs1DForOutWhenUnconnected=off
  wires:
  Data In/1 -> Data Out/1

== system bpsk_receiver/BPSK System/RF-DAC/QMC Threshold ==
  Data In : Inport
  Data Out : Outport  VectorParamsAs1DForOutWhenUnconnected=off
  wires:
  Data In/1 -> Data Out/1

== system bpsk_receiver/BPSK System/RF-DAC/RF-DAC ==
  Data In : Inport
  Cast To Double : DataTypeConversion  OutDataTypeStr=double
  Rate Transition : RateTransition  OutPortSampleTime=0
  Unbuffer : Unbuffer
  Data Out : Outport  VectorParamsAs1DForOutWhenUnconnected=off
  wires:
  Cast To Double/1 -> Rate Transition/1
  Unbuffer/1 -> Cast To Double/1
  Data In/1 -> Unbuffer/1
  Rate Transition/1 -> Data Out/1

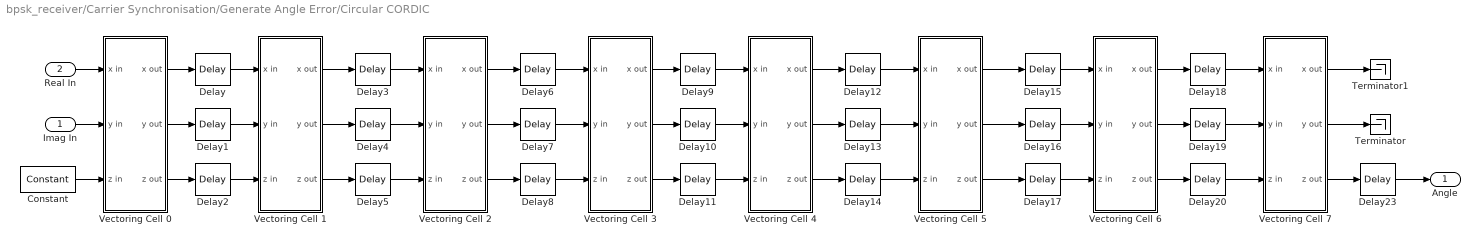
== system bpsk_receiver/Carrier Synchronisation/Generate Angle Error/Circular CORDIC ==
  Imag In : Inport
  Real In : Inport  Port=2
  Constant : xbsIndex_r4/Constant  const=0  gui_display_data_type=Fixed-point  arith_type=Signed (2's comp)  n_bits=16  bin_pt=14  preci_type=Single  exp_width=8  frac_width=24  explicit_period=off  period=1  equ=P=C  opselect=C  inp2=PCIN>>17  opr=+  inp1=P  carry=CIN  dbl_ovrd=off  block_type=constant
  Delay{,1..20,23} (22 alike) : xbsIndex_r4/Delay  rst=off  infoeditControl=Selection of Reset will increase slice count due to use of real FFs and instead of SRLs  en=off  latency=1  reg_retiming=off  dbl_ovrd=off  block_type=delay
  Terminator : Terminator
  Terminator1 : Terminator
  Vectoring Cell 0 : Subsystem  mask(Cordic Vectoring Cell){i=0}
      mask prompts: i "Iteration:"
      mask help: some notes to go here
      mask DialogControl DescGroupVar Prompt: CORDIC Vectoring Cell
      mask DialogControl DescTextVar Prompt: A single cell of a vectoring CORDIC unrolled architecture.
      mask DialogControl ParameterGroupVar Prompt: Main
  Vectoring Cell 1 : Subsystem  mask(Cordic Vectoring Cell){i=1}
      mask prompts: i "Iteration:"
      mask help: some notes to go here
      mask DialogControl DescGroupVar Prompt: CORDIC Vectoring Cell
      mask DialogControl DescTextVar Prompt: A single cell of a vectoring CORDIC unrolled architecture.
      mask DialogControl ParameterGroupVar Prompt: Main
  Vectoring Cell 2 : Subsystem  mask(Cordic Vectoring Cell){i=2}
      mask prompts: i "Iteration:"
      mask help: some notes to go here
      mask DialogControl DescGroupVar Prompt: CORDIC Vectoring Cell
      mask DialogControl DescTextVar Prompt: A single cell of a vectoring CORDIC unrolled architecture.
      mask DialogControl ParameterGroupVar Prompt: Main
  Vectoring Cell 3 : Subsystem  mask(Cordic Vectoring Cell){i=3}
      mask prompts: i "Iteration:"
      mask help: some notes to go here
      mask DialogControl DescGroupVar Prompt: CORDIC Vectoring Cell
      mask DialogControl DescTextVar Prompt: A single cell of a vectoring CORDIC unrolled architecture.
      mask DialogControl ParameterGroupVar Prompt: Main
  Vectoring Cell 4 : Subsystem  mask(Cordic Vectoring Cell){i=4}
      mask prompts: i "Iteration:"
      mask help: some notes to go here
      mask DialogControl DescGroupVar Prompt: CORDIC Vectoring Cell
      mask DialogControl DescTextVar Prompt: A single cell of a vectoring CORDIC unrolled architecture.
      mask DialogControl ParameterGroupVar Prompt: Main
  Vectoring Cell 5 : Subsystem  mask(Cordic Vectoring Cell){i=5}
      mask prompts: i "Iteration:"
      mask help: some notes to go here
      mask DialogControl DescGroupVar Prompt: CORDIC Vectoring Cell
      mask DialogControl DescTextVar Prompt: A single cell of a vectoring CORDIC unrolled architecture.
      mask DialogControl ParameterGroupVar Prompt: Main
  Vectoring Cell 6 : Subsystem  mask(Cordic Vectoring Cell){i=6}
      mask prompts: i "Iteration:"
      mask help: some notes to go here
      mask DialogControl DescGroupVar Prompt: CORDIC Vectoring Cell
      mask DialogControl DescTextVar Prompt: A single cell of a vectoring CORDIC unrolled architecture.
      mask DialogControl ParameterGroupVar Prompt: Main
  Vectoring Cell 7 : Subsystem  mask(Cordic Vectoring Cell){i=7}
      mask prompts: i "Iteration:"
      mask help: some notes to go here
      mask DialogControl DescGroupVar Prompt: CORDIC Vectoring Cell
      mask DialogControl DescTextVar Prompt: A single cell of a vectoring CORDIC unrolled architecture.
      mask DialogControl ParameterGroupVar Prompt: Main
  Angle : Outport  VectorParamsAs1DForOutWhenUnconnected=off
  wires:
  Vectoring Cell 6/3(z out) -> Delay20/1
  Delay5/1 -> Vectoring Cell 2/3(z in)
  Vectoring Cell 6/2(y out) -> Delay19/1
  Vectoring Cell 2/1(x out) -> Delay6/1
  Vectoring Cell 1/3(z out) -> Delay5/1
  Delay14/1 -> Vectoring Cell 5/3(z in)
  Delay20/1 -> Vectoring Cell 7/3(z in)
  Delay15/1 -> Vectoring Cell 6/1(x in)
  Delay7/1 -> Vectoring Cell 3/2(y in)
  Delay1/1 -> Vectoring Cell 1/2(y in)
  Vectoring Cell 3/1(x out) -> Delay9/1
  Delay13/1 -> Vectoring Cell 5/2(y in)
  Delay9/1 -> Vectoring Cell 4/1(x in)
  Vectoring Cell 1/1(x out) -> Delay3/1
  Delay16/1 -> Vectoring Cell 6/2(y in)
  Delay18/1 -> Vectoring Cell 7/1(x in)
  Vectoring Cell 0/3(z out) -> Delay2/1
  Delay10/1 -> Vectoring Cell 4/2(y in)
  Vectoring Cell 2/2(y out) -> Delay7/1
  Vectoring Cell 3/3(z out) -> Delay11/1
  Delay6/1 -> Vectoring Cell 3/1(x in)
  Delay19/1 -> Vectoring Cell 7/2(y in)
  Delay4/1 -> Vectoring Cell 2/2(y in)
  Delay3/1 -> Vectoring Cell 2/1(x in)
  Vectoring Cell 4/3(z out) -> Delay14/1
  Delay8/1 -> Vectoring Cell 3/3(z in)
  Vectoring Cell 3/2(y out) -> Delay10/1
  Vectoring Cell 1/2(y out) -> Delay4/1
  Vectoring Cell 5/1(x out) -> Delay15/1
  Delay/1 -> Vectoring Cell 1/1(x in)
  Vectoring Cell 5/2(y out) -> Delay16/1
  Vectoring Cell 0/1(x out) -> Delay/1
  Vectoring Cell 2/3(z out) -> Delay8/1
  Vectoring Cell 6/1(x out) -> Delay18/1
  Vectoring Cell 0/2(y out) -> Delay1/1
  Delay12/1 -> Vectoring Cell 5/1(x in)
  Vectoring Cell 4/2(y out) -> Delay13/1
  Vectoring Cell 4/1(x out) -> Delay12/1
  Delay2/1 -> Vectoring Cell 1/3(z in)
  Vectoring Cell 5/3(z out) -> Delay17/1
  Delay17/1 -> Vectoring Cell 6/3(z in)
  Delay11/1 -> Vectoring Cell 4/3(z in)
  Vectoring Cell 7/3(z out) -> Delay23/1
  Real In/1 -> Vectoring Cell 0/1(x in)
  Imag In/1 -> Vectoring Cell 0/2(y in)
  Constant/1 -> Vectoring Cell 0/3(z in)
  Delay23/1 -> Angle/1
  Vectoring Cell 7/2(y out) -> Terminator/1
  Vectoring Cell 7/1(x out) -> Terminator1/1

== system bpsk_receiver/Carrier Synchronisation/Generate NCO/Loop Filter ==
  note: The input to the loop filter should only be changed once per symbol.
      |
      | Use an enable register with the strobe from the NCC to hold the data in place.
  Signal : Inport
  Strobe : Inport  Port=2
  Reset : Inport  Port=3
  AddSub : xbsIndex_r4/AddSub  mode=Addition  use_carryin=off  use_carryout=off  en=off  latency=0  precision=User Defined  arith_type="Signed  (2's comp)"  n_bits=36  bin_pt=34  quantization=Truncate  overflow=Flag as error  use_behavioral_HDL=off  hw_selection=Fabric  pipelined=off  dbl_ovrd=off  block_type=addsub
  AddSub1 : xbsIndex_r4/AddSub  mode=Addition  use_carryin=off  use_carryout=off  en=off  latency=0  precision=Full  arith_type="Signed  (2's comp)"  n_bits=32  bin_pt=31  quantization=Truncate  overflow=Wrap  use_behavioral_HDL=off  hw_selection=Fabric  pipelined=off  dbl_ovrd=off  block_type=addsub
  K1_Gain : xbsIndex_r4/CMult  const=K1  gui_display_data_type=Fixed-point  const_n_bits=16  const_bin_pt=16  float_type=Single  exp_bits=8  fraction_bits=24  en=off  latency=0  precision=Full  arith_type="Signed  (2's comp)"  n_bits=20  bin_pt=14  quantization=Truncate  overflow=Wrap  use_behavioral_HDL=off  mem_type=Distributed RAM  pipeline=off  dbl_ovrd=off  block_type=cmult
  K2_Gain : xbsIndex_r4/CMult  const=K2  gui_display_data_type=Fixed-point  const_n_bits=16  const_bin_pt=16  float_type=Single  exp_bits=8  fraction_bits=24  en=off  latency=0  precision=Full  arith_type="Signed  (2's comp)"  n_bits=20  bin_pt=14  quantization=Truncate  overflow=Wrap  use_behavioral_HDL=off  mem_type=Distributed RAM  pipeline=off  dbl_ovrd=off  block_type=cmult
  Register : xbsIndex_r4/Register  init=0  rst=on  en=on  dbl_ovrd=off  block_type=register
  Register1 : xbsIndex_r4/Register  init=0  rst=on  en=on  dbl_ovrd=off  block_type=register
  Register3 : xbsIndex_r4/Register  init=0  rst=off  en=off  dbl_ovrd=off  block_type=register
  Register4 : xbsIndex_r4/Register  init=0  rst=off  en=off  dbl_ovrd=off  block_type=register
  Error : Outport  VectorParamsAs1DForOutWhenUnconnected=off
  Valid : Outport  Port=2  VectorParamsAs1DForOutWhenUnconnected=off
  wires:
  Reset/1 -> Register/2, Register1/2
  Signal/1 -> Register1/1
  K2_Gain/1 -> AddSub/1
  AddSub/1 -> AddSub1/2, Register/1
  Register/1 -> AddSub/2
  Register1/1 -> K2_Gain/1, K1_Gain/1
  AddSub1/1 -> Register3/1
  K1_Gain/1 -> AddSub1/1
  Register3/1 -> Error/1
  Register4/1 -> Valid/1
  Strobe/1 -> Register4/1, Register/3, Register1/3

== system bpsk_receiver/Carrier Synchronisation/Generate NCO/NCO ==
  Step Size : Inport
  En_in : Inport  Port=2
  AddSub4 : xbsIndex_r4/AddSub  mode=Addition  use_carryin=off  use_carryout=off  en=off  latency=0  precision=User Defined  arith_type="Signed  (2's comp)"  n_bits=n+b  bin_pt=b  quantization=Truncate  overflow=Wrap  use_behavioral_HDL=off  hw_selection=Fabric  pipelined=off  dbl_ovrd=off  block_type=addsub
  CMult1 : xbsIndex_r4/CMult  const=(2^n)/(2*pi)  gui_display_data_type=Fixed-point  const_n_bits=k_n+b  const_bin_pt=b  float_type=Single  exp_bits=8  fraction_bits=24  en=off  latency=0  precision=User Defined  arith_type="Signed  (2's comp)"  n_bits=n+b  bin_pt=b  quantization=Truncate  overflow=Wrap  use_behavioral_HDL=off  mem_type=Distributed RAM  pipeline=off  dbl_ovrd=off  block_type=cmult
  Convert1 : xbsIndex_r4/Convert  gui_display_data_type=Fixed-point  arith_type=Unsigned  n_bits=n  bin_pt=0  float_type=Single  exp_bits=8  fraction_bits=24  quantization=Truncate  overflow=Wrap  en=off  latency=0  pipeline=off  dbl_ovrd=off  block_type=convert
  Cos ROM : xbsIndex_r4/ROM  depth=2^n  initVector=cos(pi*(0:((2^n)-1))/(2^(n-1)))  distributed_mem=Block RAM  rst=off  init_reg=0  en=off  latency=1  gui_display_data_type=Fixed-point  arith_type="Signed  (2's comp)"  n_bits=16  bin_pt=14  preci_type=Single  exp_width=8  frac_width=24  optimize=Area  use_rpm=on  dbl_ovrd=off  simulation_type=fast_sim  block_type=sprom
  Neg Sin ROM : xbsIndex_r4/ROM  depth=2^n  initVector=-sin(pi*(0:((2^n)-1))/(2^(n-1)))  distributed_mem=Block RAM  rst=off  init_reg=0  en=off  latency=1  gui_display_data_type=Fixed-point  arith_type="Signed  (2's comp)"  n_bits=16  bin_pt=14  preci_type=Single  exp_width=8  frac_width=24  optimize=Area  use_rpm=on  dbl_ovrd=off  simulation_type=fast_sim  block_type=sprom
  Register : xbsIndex_r4/Register  init=0  rst=off  en=off  dbl_ovrd=off  block_type=register
  Register1 : xbsIndex_r4/Register  init=0  rst=off  en=on  dbl_ovrd=off  block_type=register
  Cos : Outport  VectorParamsAs1DForOutWhenUnconnected=off
  Neg Sin : Outport  Port=2  VectorParamsAs1DForOutWhenUnconnected=off
  En_out : Outport  Port=3  VectorParamsAs1DForOutWhenUnconnected=off
  wires:
  Convert1/1 -> Neg Sin ROM/1, Cos ROM/1
  AddSub4/1 -> Register1/1, Convert1/1
  Neg Sin ROM/1 -> Neg Sin/1
  Register1/1 -> AddSub4/2
  CMult1/1 -> AddSub4/1
  Step Size/1 -> CMult1/1
  En_in/1 -> Register/1, Register1/2
  Cos ROM/1 -> Cos/1
  Register/1 -> En_out/1

== system bpsk_receiver/Frame Synchronisation/Frame Sync/DBPSK Convert ==
  Data In : Inport
  Valid In : Inport  Port=2
  Constant : xbsIndex_r4/Constant  const=1.0  gui_display_data_type=Fixed-point  arith_type=Signed (2's comp)  n_bits=2  bin_pt=0  preci_type=Single  exp_width=8  frac_width=24  explicit_period=off  period=1  equ=P=C  opselect=C  inp2=PCIN>>17  opr=+  inp1=P  carry=CIN  dbl_ovrd=off  block_type=constant
  Constant1 : xbsIndex_r4/Constant  const=-1.0  gui_display_data_type=Fixed-point  arith_type=Signed (2's comp)  n_bits=2  bin_pt=0  preci_type=Single  exp_width=8  frac_width=24  explicit_period=off  period=1  equ=P=C  opselect=C  inp2=PCIN>>17  opr=+  inp1=P  carry=CIN  dbl_ovrd=off  block_type=constant
  Mux : xbsIndex_r4/Mux  inputs=2  en=off  latency=0  precision=Full  arith_type=Unsigned  n_bits=16  bin_pt=14  quantization=Truncate  overflow=Wrap  dbl_ovrd=off  block_type=mux
  Data Out : Outport  VectorParamsAs1DForOutWhenUnconnected=off
  Valid Out : Outport  Port=2  VectorParamsAs1DForOutWhenUnconnected=off
  wires:
  Constant/1 -> Mux/2
  Constant1/1 -> Mux/3
  Mux/1 -> Data Out/1
  Valid In/1 -> Valid Out/1
  Data In/1 -> Mux/1

== system bpsk_receiver/Frame Synchronisation/Frame Sync/DBPSK Decision ==
  Data In : Inport
  Valid In : Inport  Port=2
  Logical1 : xbsIndex_r4/Logical  logical_function=XOR  inputs=2  en=off  latency=0  precision=Full  arith_type=Unsigned  n_bits=16  bin_pt=0  align_bp=on  dbl_ovrd=off  block_type=logical
  Register : xbsIndex_r4/Register  init=0  rst=off  en=on  dbl_ovrd=off  block_type=register
  Register2 : xbsIndex_r4/Register  init=0  rst=off  en=off  dbl_ovrd=off  block_type=register
  Register3 : xbsIndex_r4/Register  init=0  rst=off  en=on  dbl_ovrd=off  block_type=register
  Register4 : xbsIndex_r4/Register  init=0  rst=off  en=on  dbl_ovrd=off  block_type=register
  Register5 : xbsIndex_r4/Register  init=0  rst=off  en=off  dbl_ovrd=off  block_type=register
  Data Out : Outport  VectorParamsAs1DForOutWhenUnconnected=off
  Valid Out : Outport  Port=2  VectorParamsAs1DForOutWhenUnconnected=off
  wires:
  Register4/1 -> Data Out/1
  Register2/1 -> Register4/2, Register5/1, Register3/2
  Logical1/1 -> Register4/1
  Register/1 -> Logical1/2, Register3/1
  Register3/1 -> Logical1/1
  Valid In/1 -> Register2/1, Register/2
  Register5/1 -> Valid Out/1
  Data In/1 -> Register/1

== system bpsk_receiver/Frame Synchronisation/Frame Sync/Rising Edge Detector ==
  Input : Inport
  Inverter : xbsIndex_r4/Inverter  en=off  latency=0  dbl_ovrd=off  block_type=inv
  Logical1 : xbsIndex_r4/Logical  logical_function=AND  inputs=2  en=off  latency=0  precision=Full  arith_type=Unsigned  n_bits=16  bin_pt=0  align_bp=on  dbl_ovrd=off  block_type=logical
  Register2 : xbsIndex_r4/Register  init=0  rst=off  en=off  dbl_ovrd=off  block_type=register
  Output : Outport  VectorParamsAs1DForOutWhenUnconnected=off
  wires:
  Logical1/1 -> Output/1
  Input/1 -> Logical1/2, Register2/1
  Inverter/1 -> Logical1/1
  Register2/1 -> Inverter/1
